simulink model "Block_TF_SS"  (R2014b)
settings: Solver=ode45  StartTime=0.0  StopTime=10.0  RelTol=1e-3
settings Model: Creator=99641  LastModifiedBy=99641

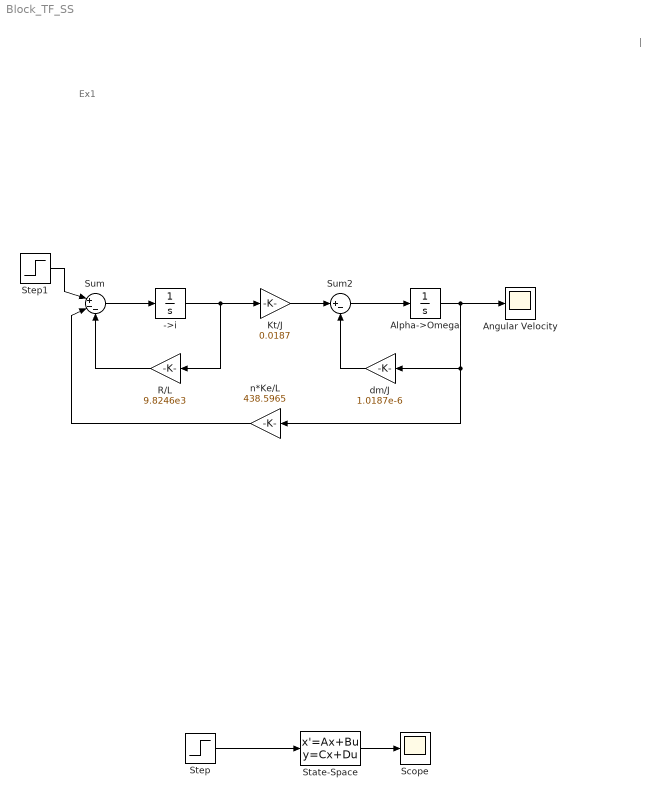
== system Block_TF_SS ==
  note: |
  note: Ex1
  ->i : Integrator
  Alpha->Omega : Integrator
  Angular Velocity : Scope
  Kt/J : Gain  Gain=0.0187
  R/L : Gain  Gain=9.8246e3
  Scope : Scope
      settings: SaveName=ScopeData2
  State-Space : StateSpace  A=[0,0,-22.4;0,0,0.0187;0,0,0]  B=[0.2;0;0]  C=[1,0,0;0,1,0]  D=[0;0]  X0=0
  Step : Step  SampleTime=0
  Step1 : Step  SampleTime=0
  Sum : Sum  Inputs=|+--
  Sum2 : Sum  Inputs=|+-
  dm/J : Gain  Gain=1.0187e-6
  n*Ke/L : Gain  Gain=438.5965
  wires:
  State-Space/1 -> Scope/1
  Step/1 -> State-Space/1
  Sum/1 -> ->i/1
  ->i/1 -> R/L/1, Kt/J/1
  Kt/J/1 -> Sum2/1
  Sum2/1 -> Alpha->Omega/1
  R/L/1 -> Sum/3
  n*Ke/L/1 -> Sum/2
  dm/J/1 -> Sum2/2
  Alpha->Omega/1 -> Angular Velocity/1, n*Ke/L/1, dm/J/1
  Step1/1 -> Sum/1
